simulink model "rough"  (R2023b)
settings: Solver=FixedStepAuto  StartTime=0.0  StopTime=inf  RelTol=1e-3
undefined symbols (not defined in the file): CoordinateFrame, TypeMask, Velocity, YawRate
libraries: robotlib x2, mpclib x1, aerolibanimutils x1
settings Model: SimulationMode=external  Creator=oem  LastModifiedBy=farhan
settings OptimizationCC: EnhancedBackFolding=on  PassReuseOutputArgsAs=Individual arguments  ZeroExternalMemoryAtStartup=off  ZeroInternalMemoryAtStartup=off  MaxStackSize=64  OptimizeBlockOrder=speed  DifferentSizesBufferReuse=on  OptimizationCustomize=off  EfficientTunableParamExpr=on
settings DebuggingCC: ParameterTunabilityLossMsg=error
settings HardwareCC: ProdBitPerPointer=32  ProdBitPerSizeT=32  ProdBitPerPtrDiffT=32  ProdLargestAtomicFloat=None  ProdIntDivRoundTo=Undefined  ProdEndianess=Unspecified  ProdWordSize=32  ProdHWDeviceType=Generic->Unspecified (assume 32-bit Generic)
settings SFSimCC: MATLABDynamicMemAlloc=off
settings RTWCC: Description=Embedded Coder  SystemTargetFile=ert.tlc  HardwareBoard=Robot Operating System (ROS)  TLCOptions="-aInlineSetEventsForThisBaseRateFcn=TLC_FALSE -aSuppressMultiTaskScheduler=TLC_FALSE  -aRateBasedStepFcn=0"  TemplateMakefile=ert_default_tmf  Toolchain=Catkin  TargetLang=C++
settings CodeAppCC: ForceParamTrailComments=on  IgnoreCustomStorageClasses=off  OperatorAnnotations=on  SimulinkDataObjDesc=on  SFDataObjDesc=on  InsertBlockDesc=on
settings ERTTargetCC: SupportContinuousTime=on  SupportVariableSizeSignals=on  ExtMode=on  ExtModeMexArgs='127.0.0.1' 0 17725

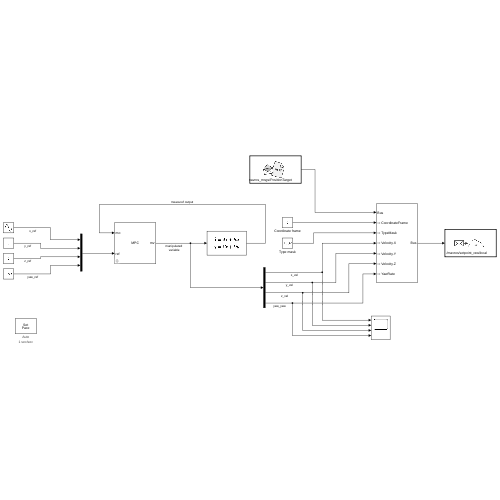
[thumbnail: Simulink's stored preview of the top-level diagram]
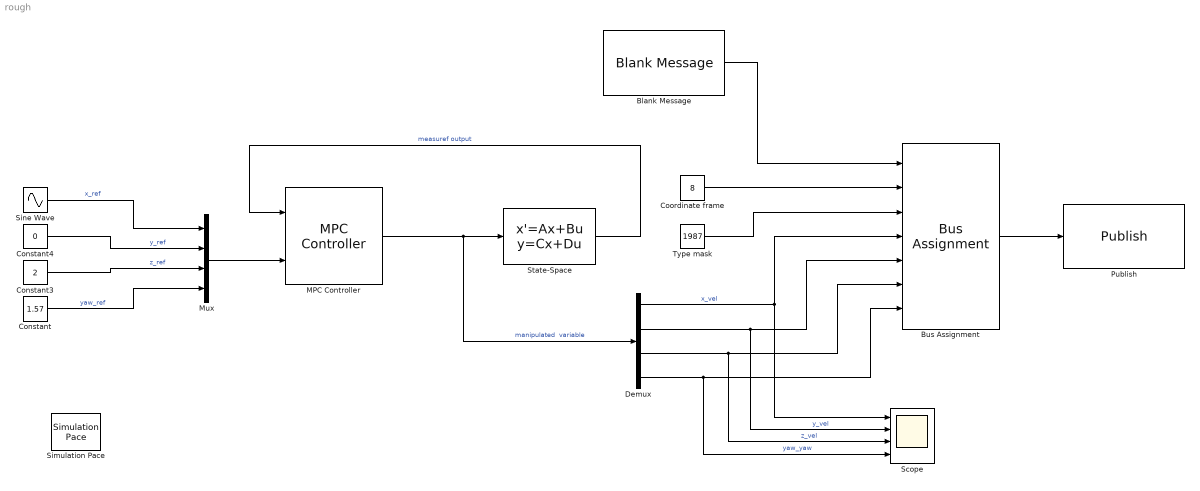
== system rough ==
  Blank Message : robotlib/Blank Message  messageClass=Message  entityType=mavros_msgs/PositionTarget  messageType=mavros_msgs/PositionTarget  SampleTime=inf  legacyBusStruct=off
  Bus Assignment : BusAssignment  AssignedSignals=CoordinateFrame,TypeMask,Velocity.X,Velocity.Y,Velocity.Z,YawRate
  Constant : Constant  Value=1.57
  Constant3 : Constant  Value=2
  Constant4 : Constant  Value=0
  Coordinate frame : Constant  Value=8  OutDataTypeStr=uint8
  Demux : Demux
  MPC Controller : mpclib/MPC Controller  SCDEnableBlockLinearizationSpecification=on  mpcobj=mpc1  is_multiple=0  enable_value=0  return_u0=off  updateMPCinCallerWorkspace=on  md_inport=off  mv_inport=off  uref_inport=off  return_cost=off  return_mvseq=off  return_qpstatus=off  return_xseq=off  return_state=off  return_ovseq=off  state_inport=off  umin_inport=off  umax_inport=off  ymin_inport=off  ymax_inport=off  cc_inport=off  ywt_inport=off  uwt_inport=off  duwt_inport=off  rhoeps_inport=off  pm_inport=off  MaximumP=10  HorizonChoice=FixedHorizon  n_ts=0.1  n_p=20  n_mv=4  n_md=0  n_ud=0  n_mo=4  n_uo=0  BlockDataType=double  SampleTimeInherited=off  switch_inport=off
  Mux : Mux
  Publish : robotlib/Publish  topicSource=Specify your own  topic=/mavros/setpoint_raw/local  messageType=mavros_msgs/PositionTarget  legacyBusStruct=off  messageQueueLength=1
  Scope : Scope  NumInputPorts=4
  Simulation Pace : aerolibanimutils/Simulation Pace  SimulationPace=1  SleepMode=Auto  OutputPaceError=off  SampleTime=1/30
  Sine Wave : Sin  SampleTime=0
  State-Space : StateSpace  A=zeros(4, 4)  B=eye(4, 4)  C=eye(4, 4)  D=zeros(4, 4)  InitialCondition=[0, 0, 2, 1.57]  ContinuousStateAttributes='position'
  Type mask : Constant  Value=1987  OutDataTypeStr=uint16
  wires:
  MPC Controller/1 -> Demux/1, State-Space/1  "manipulated  variable"
  Bus Assignment/1 -> Publish/1
  Blank Message/1 -> Bus Assignment/1
  State-Space/1 -> MPC Controller/1  "measuref output"
  Demux/1 -> Scope/1, Bus Assignment/4  "x_vel"
  Demux/2 -> Scope/2, Bus Assignment/5  "y_vel"
  Demux/3 -> Scope/3, Bus Assignment/6  "z_vel"
  Demux/4 -> Scope/4, Bus Assignment/7  "yaw_yaw"
  Coordinate frame/1 -> Bus Assignment/2
  Type mask/1 -> Bus Assignment/3
  Mux/1 -> MPC Controller/2
  Sine Wave/1 -> Mux/1  "x_ref"
  Constant4/1 -> Mux/2  "y_ref"
  Constant3/1 -> Mux/3  "z_ref"
  Constant/1 -> Mux/4  "yaw_ref"
